simulink model "single_tank_linear_real_PID"  (R2022a)
settings: Solver=VariableStepAuto  StartTime=0.0  StopTime=10.0  RelTol=1e-3
values from neighbouring files (symbols this model uses):
  h_0 = 30    [state_space_models.m]
  I_0 = [ 0 0 0 ]    [state_space_models.m]
  MPC_active = 1    [run_simulation_noise.m]    (also in run_simulation_smooth.m)
  noise = 0    [run_simulation_model_errors.m]    (also in run_simulation_noise.m = 1; run_simulation_smooth.m)
  sys_kd = c2d(ss(A_kc,B_kc,C_kc,D_kc), dt)    [state_space_models.m]
  sys_pd = c2d(ss(A_pc,[B_pc B_pc_d],C_pc,D_pc), dt)    [state_space_models.m]
  u_0 = 60    [state_space_models.m]
  x_0 = 0    [state_space_models.m]
undefined symbols (not defined in the file or in its folder): dist, dt, K_noise, K_white
libraries: mpclib x1, simulink x1
settings Model: Creator=100238  LastModifiedBy=100238

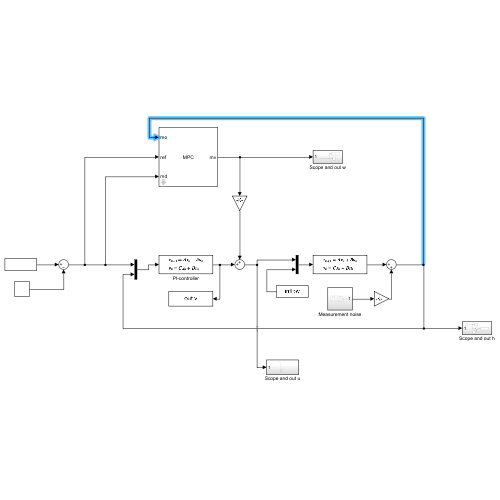
[thumbnail: Simulink's stored preview of the top-level diagram]
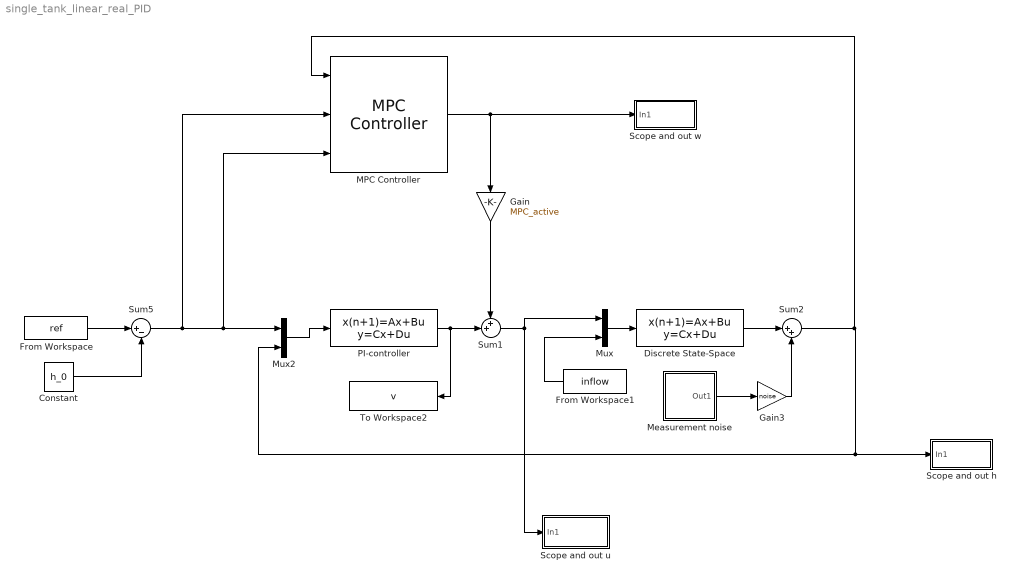
== system single_tank_linear_real_PID ==
  Constant : Constant  Value=h_0
  Discrete State-Space : DiscreteStateSpace  A=sys_pd.A  B=sys_pd.B  C=sys_pd.C  D=sys_pd.D  InitialCondition=x_0  SampleTime=dt
  From Workspace : FromWorkspace  VariableName=ref  SampleTime=dt
  From Workspace1 : FromWorkspace  VariableName=inflow  SampleTime=dt
  Gain : Gain  Gain=MPC_active
  Gain3 : Gain  Gain=noise
  MPC Controller : mpclib/MPC Controller  SCDEnableBlockLinearizationSpecification=on  mpcobj=mpc_controller  is_multiple=0  enable_value=0  return_u0=off  updateMPCinCallerWorkspace=on  md_inport=on  mv_inport=off  uref_inport=off  return_cost=off  return_mvseq=off  return_qpstatus=off  return_xseq=off  return_state=off  return_ovseq=off  state_inport=off  umin_inport=off  umax_inport=off  ymin_inport=off  ymax_inport=off  cc_inport=off  ywt_inport=off  uwt_inport=off  duwt_inport=off  rhoeps_inport=off  pm_inport=off  MaximumP=10  HorizonChoice=FixedHorizon  n_ts=1  n_p=150  n_mv=1  n_md=1  n_ud=0  n_mo=1  n_uo=0  BlockDataType=double  SampleTimeInherited=off  switch_inport=off
  Measurement noise : Subsystem
  Mux : Mux  Inputs=2
  Mux2 : Mux  Inputs=2
  PI-controller : DiscreteStateSpace  A=sys_kd.A  B=sys_kd.B  C=sys_kd.C  D=sys_kd.D  InitialCondition=I_0  SampleTime=dt
  Scope and out h : Subsystem
  Scope and out u : Subsystem
  Scope and out w : Subsystem
  Sum1 : Sum  Inputs=++|
  Sum2 : Sum  Inputs=|++
  Sum5 : Sum  Inputs=|+-
  To Workspace2 : ToWorkspace  VariableName=v  SampleTime=dt
  wires:
  From Workspace1/1 -> Mux/2
  PI-controller/1 -> Sum1/2, To Workspace2/1
  Sum1/1 -> Scope and out u/1(In1), Mux/1
  MPC Controller/1 -> Gain/1, Scope and out w/1(In1)
  From Workspace/1 -> Sum5/1
  Constant/1 -> Sum5/2
  Mux/1 -> Discrete State-Space/1
  Measurement noise/1(Out1) -> Gain3/1
  Discrete State-Space/1 -> Sum2/1
  Sum5/1 -> MPC Controller/2, Mux2/1, MPC Controller/3
  Mux2/1 -> PI-controller/1
  Gain/1 -> Sum1/1
  Sum2/1 -> MPC Controller/1, Mux2/2, Scope and out h/1(In1)
  Gain3/1 -> Sum2/2

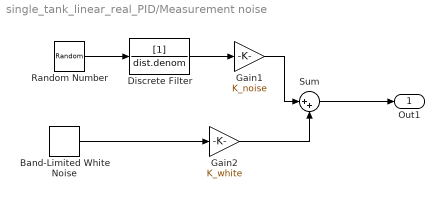
== system single_tank_linear_real_PID/Measurement noise ==
  Band-Limited White Noise : simulink/Sources/Band-Limited White Noise  Cov=[0.03]  Ts=dt  seed=[23341]
  Discrete Filter : DiscreteFilter  Denominator=dist.denom  SampleTime=dt
  Gain1 : Gain  Gain=K_noise
  Gain2 : Gain  Gain=K_white
  Random Number : RandomNumber  Seed=1  SampleTime=dt
  Sum : Sum  Inputs=|++
  Out1 : Outport
  wires:
  Random Number/1 -> Discrete Filter/1
  Gain1/1 -> Sum/1
  Discrete Filter/1 -> Gain1/1
  Sum/1 -> Out1/1
  Band-Limited White Noise/1 -> Gain2/1
  Gain2/1 -> Sum/2

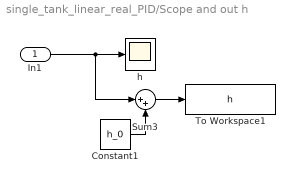
== system single_tank_linear_real_PID/Scope and out h ==
  In1 : Inport
  Constant1 : Constant  Value=h_0
  Sum3 : Sum  Inputs=|++
  To Workspace1 : ToWorkspace  VariableName=h  SampleTime=dt
  h : Scope
  wires:
  Constant1/1 -> Sum3/2
  Sum3/1 -> To Workspace1/1
  In1/1 -> Sum3/1, h/1

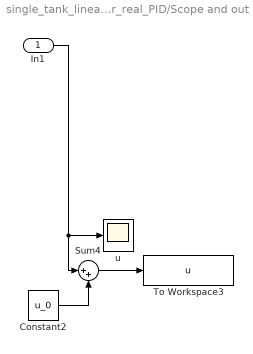
== system single_tank_linear_real_PID/Scope and out u ==
  In1 : Inport
  Constant2 : Constant  Value=u_0
  Sum4 : Sum  Inputs=|++
  To Workspace3 : ToWorkspace  VariableName=u  SampleTime=dt
  u : Scope
  wires:
  Constant2/1 -> Sum4/2
  In1/1 -> u/1, Sum4/1
  Sum4/1 -> To Workspace3/1

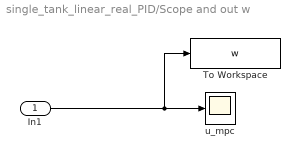
== system single_tank_linear_real_PID/Scope and out w ==
  In1 : Inport
  To Workspace : ToWorkspace  VariableName=w  SampleTime=dt
  u_mpc : Scope
  wires:
  In1/1 -> To Workspace/1, u_mpc/1
